simulink library "thc"  (R2021b)
settings: Solver=VariableStepAuto  StartTime=0.0  StopTime=10.0  RelTol=1e-3
undefined symbols (not defined in the file or in its folder): ATHC_APTCQA_X_C, ATHC_APTCQB_X_C, ATHC_dAy_X_C, ATHC_Qeq_X_kmh, ATHC_VbaseC_X_C, ATHC_VbaseC_Y_W, ATHC_VbaseD_X_C, ATHC_VbaseH_X_C, FALSE, KTHC_ACMaxMinT_sec, KTHC_aDeice_K, KTHC_AGSDefLv_K, KTHC_AGSLv1_K, KTHC_AGSLv2_K, KTHC_AGSLv3_K, KTHC_AGSLv4_K, KTHC_AGSLv5_K, KTHC_AirIntUpdateT_sec, KTHC_APTCOneZoneMax_W, KTHC_APTCQMaxC_W, KTHC_APTCQminC_W, KTHC_APTCQminD_W, KTHC_APTCQminRe1_W, KTHC_APTCQminRe_W, KTHC_APTCQoffT_cnt, KTHC_APTCQonT_cnt, KTHC_APTCRiLeMaxDff_W, KTHC_APTCRiLeMinDff_W, KTHC_BatInTempDef_C, KTHC_bDeice_K, KTHC_CompMaxDeice_rpm, KTHC_CompMinDeice_rpm, KTHC_CompSotxvOp_K, KTHC_CompSotxvOpLow_rpm, KTHC_CompSpdmax_rpm, KTHC_CompSpdmaxBC1_rpm, KTHC_CompSpdmaxBC_rpm, KTHC_CompSpdmid1_rpm, KTHC_CompSpdmid2_rpm, KTHC_CompSpdmid3_rpm, KTHC_CompSpdmid_rpm, KTHC_CompSpdmin_rpm, KTHC_DAPTCQ1_W, KTHC_DAPTCQ2_W, KTHC_DAPTCQ3_W, KTHC_DcChSetTemp_C, KTHC_DehumidityEN_flg, KTHC_DeiceCycTime_K, KTHC_DTambSat1_C, KTHC_DTambSat2_C, KTHC_DTambsat3_C, KTHC_DTambsat4_C, KTHC_DTambSat5_C, KTHC_DTambSat_C, KTHC_DTcabin10_C, KTHC_DTCabin11_C, KTHC_DTcabin12_C, KTHC_DTcabin1_C, KTHC_DTcabin2_C, KTHC_DTcabin3_C ... (+347)
libraries: simulink x80
(part 1 of 8)
settings Model: Creator=FVT20341  LastModifiedBy=FVT22063

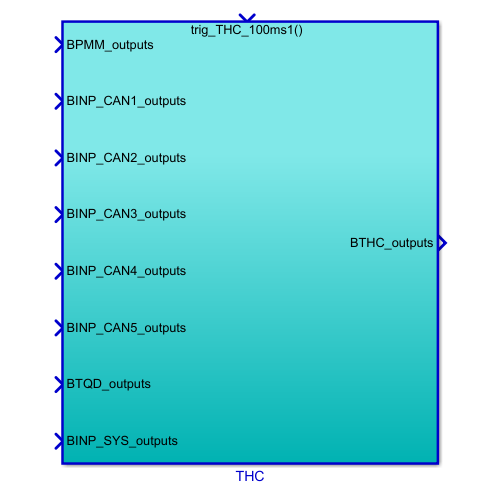
[thumbnail: Simulink's stored preview of the top-level diagram]
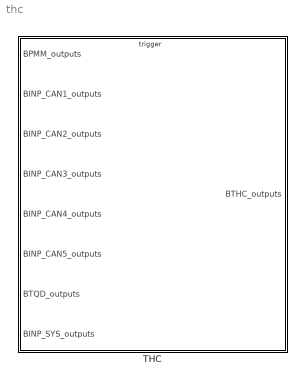
== system thc ==
  THC : Subsystem  TreatAsAtomicUnit=on
      settings: RTWSystemCode=Nonreusable function  RTWFcnNameOpts=Use subsystem name  RTWFileNameOpts=Use subsystem name

== system thc/THC ==
  BPMM_outputs : Inport  OutDataTypeStr=Bus: BPMM_outputs
  BINP_CAN1_outputs : Inport  Port=2  OutDataTypeStr=Bus: BINP_CAN1_outputs
  BINP_CAN2_outputs : Inport  Port=3  OutDataTypeStr=Bus: BINP_CAN2_outputs
  BINP_CAN3_outputs : Inport  Port=4  OutDataTypeStr=Bus: BINP_CAN3_outputs
  BINP_CAN4_outputs : Inport  Port=5  OutDataTypeStr=Bus: BINP_CAN4_outputs
  BINP_CAN5_outputs : Inport  Port=6  OutDataTypeStr=Bus: BINP_CAN5_outputs
  BTQD_outputs : Inport  Port=7  OutDataTypeStr=Bus: BTQD_outputs
  BINP_SYS_outputs : Inport  Port=8  OutDataTypeStr=Bus: BINP_SYS_outputs
  trig_THC_100ms1 : TriggerPort  TriggerType=function-call  VariantControl=(inherit)
  Bus Creator : BusCreator  Inputs=74  OutDataTypeStr=Bus: BTHC_outputs  NonVirtualBus=on
  Bus Selector : BusSelector  OutputSignals=VINP_FlashACModeMem_enum,VINP_FlashFace_flg,VINP_FlashFoot_flg,VINP_FlashFrost_flg,VINP_FlashFaceM_flg,VINP_FlashFootM_flg,VINP_FlashCCUSyncSts_flg,VINP_FlashACForceOFF_flg,VINP_FlashsigRecircSt_flg,VINP_FlashRecAutoFlg_flg,VINP_FlashAirIntenZone1M_enum,VINP_Flashfdefog_flg,VINP_FlashsigSetTempZon1St_C,VINP_FlashsigSetTempZon2StM_C
  Bus Selector1 : BusSelector  OutputSignals=VINP_VehSpeed_kph
  Bus Selector2 : BusSelector  OutputSignals=VINP_HVBMTempMax_C,VINP_HVBMTempMin_C,VINP_OBCTemp_C,VINP_DCDCTemp_C,VINP_RrTMTemp_C,VINP_RrMCUTemp_C,VINP_FrTMTemp_C,VINP_FrMCUTemp_C,VINP_ChrgPlugSta_enum,VINP_FrLLCTemp_C,VINP_RrLLCTemp_C,VINP_HVBIsoImpedenceN_Megaohm,VINP_HVBIsoImpedenceP_Megaohm,VINP_HVBHVILErr_flg
  Bus Selector3 : BusSelector  OutputSignals=VINP_PTHighTact_C,VINP_COMPStatorSpd_rpm,VINP_CompProEN_flg,VINP_PTLowP1_KPa,VINP_PTLowT1_C,VINP_PTLowP2_KPa,VINP_PTLowT2_C,VINP_PTHighP_KPa,VINP_Tamb_C,VINP_BatInTemp_C,VINP_BatOutTemp_C,VINP_MotorInTemp_C,VINP_MotorOutTemp_C,VINP_Tincar_C,VINP_SolarL_W,VINP_SolarR_W,VINP_Tevap_C,VINP_TFaceL_C,VINP_TFaceR_C,VINP_TFootL_C,VINP_TFootR_C,VINP_TFootRr_C,VINP_TFaceRr_C,VINP_EACProtectEnable_enum,VINP_TambErr_enum,VINP_SolarLErr_enum,VINP_SolarRErr_enum,VINP_TevapErr_enum,VINP_TFaceLErr_enum,VINP_TFaceRErr_enum,VINP_TFootLErr_enum,VINP_TFootRErr_enum,VINP_TFaceRrErr_enum,VINP_TFootRrErr_enum,VINP_TincarErr_enum,VINP_BatInTempErr_enum,VINP_MotorInTempErr_enum,VINP_MotorOutTempErr_enum,VINP_FanErr_enum,VINP_AGSErr_enum,VINP_EWP3Err_enum,VINP_PTHighPErr_enum,VINP_PTHighTactErr_enum,VINP_SOV1Err_enum,VINP_SOV2Err_enum,VINP_SOV3Err_enum,VINP_EXV1Err_enum,VINP_EXV2Err_enum,VINP_COMPErr_enum,VINP_BlowerErr_enum,VINP_PTLowP1Err_enum,VINP_PTLowT1Err_enum,VINP_PTLowP2Err_enum,VINP_PTLowT2Err_enum,VINP_SOTXVErr_enum,VINP_FrntPTCRearLeActHeatPwr_W,VINP_FrntPTCRearRiActHeatPwr_W,VINP_FrntPTCRiActHeatPwr_W
  Bus Selector4 : BusSelector  OutputSignals=VINP_OFFACMODE_enum,VINP_FCPFrEvtBtnACMaxReq_flg,VINP_FCPFrEvtBtnACReq_flg,VINP_FCPFrEvtBtnAutoReq_flg,VINP_FCPFrEvtBtnSyncReq_flg,VINP_sigAirIntenZon1Req_enum,VINP_sigRecircReq_flg,VINP_sigFaceReq_flg,VINP_sigFootReq_flg,VINP_sigDfrstReq_flg,VINP_sigSetTempZon1Req_C,VINP_CANMsgValidIVI2_flg,VINP_sigSetTempZon2Req_C,VINP_SmartEcoModeSW_flg
  Bus Selector5 : BusSelector  OutputSignals=VTQD_ShiftGearPosn_enum
  Bus Selector6 : BusSelector  OutputSignals=VINP_RemoteACTemp_C,VINP_RemoteAutoReq_flg
  Bus Selector7 : BusSelector  OutputSignals=VPMM_PowerSta_enum
  Ground : Ground
  Ground1 : Ground
  ThermalControl : Subsystem
  BTHC_outputs : Outport  OutDataTypeStr=Bus: BTHC_outputs
  wires:
  BPMM_outputs/1 -> Bus Selector7/1
  Bus Selector7/1 -> ThermalControl/1(VPMM_PwrSta_enum)  "<VPMM_PowerSta_enum>"
  BINP_CAN1_outputs/1 -> Bus Selector1/1
  Bus Selector1/1 -> ThermalControl/4(VINP_VehSpeed_kph)  "<VINP_VehSpeed_kph>"
  BINP_CAN3_outputs/1 -> Bus Selector2/1
  Bus Selector2/3 -> ThermalControl/7(VINP_OBCTemp_C)  "<VINP_OBCTemp_C>"
  Bus Selector2/4 -> ThermalControl/8(VINP_DCDCTemp_C)  "<VINP_DCDCTemp_C>"
  Bus Selector2/2 -> ThermalControl/6(VINP_HVBMTempMin_C)  "<VINP_HVBMTempMin_C>"
  Bus Selector2/5 -> ThermalControl/9(VINP_RrTMTemp_C)  "<VINP_RrTMTemp_C>"
  Bus Selector2/1 -> ThermalControl/5(VINP_HVBMTempMax_C)  "<VINP_HVBMTempMax_C>"
  Bus Selector2/6 -> ThermalControl/10(VINP_RrMCUTemp_C)  "<VINP_RrMCUTemp_C>"
  Bus Selector2/7 -> ThermalControl/11(VINP_FrTMTemp_C)  "<VINP_FrTMTemp_C>"
  Bus Selector2/8 -> ThermalControl/12(VINP_FrMCUTemp_C)  "<VINP_FrMCUTemp_C>"
  ThermalControl/32(VTHC_sigClntTHvBattOut_C) -> Bus Creator/32  "VTHC_sigClntTHvBattOut_C"
  ThermalControl/31(VTHC_sigSetTempZon2St_C) -> Bus Creator/31  "VTHC_sigSetTempZon2St_C"
  ThermalControl/30(VTHC_sigSetTempZon1St_C) -> Bus Creator/30  "VTHC_sigSetTempZon1St_C"
  ThermalControl/29(VTHC_sigRecircSt_flg) -> Bus Creator/29  "VTHC_sigRecircSt_flg"
  ThermalControl/28(VTHC_sigWindDirZon1St_enum) -> Bus Creator/28  "VTHC_sigWindDirZon1St_enum"
  ThermalControl/27(VTHC_sigAirIntenZon1St_enum) -> Bus Creator/27  "VTHC_sigAirIntenZon1St_enum"
  ThermalControl/26(VTHC_CCUSyncLampSts_flg) -> Bus Creator/26  "VTHC_CCUSyncLampSts_flg"
  ThermalControl/25(VTHC_CCUACMaxLampSts_flg) -> Bus Creator/25  "VTHC_CCUACMaxLampSts_flg"
  ThermalControl/24(VTHC_CCUAutoLampSts_flg) -> Bus Creator/24  "VTHC_CCUAutoLampSts_flg"
  ThermalControl/23(VTHC_CCUACLampSts_flg) -> Bus Creator/23  "VTHC_CCUACLampSts_flg"
  ThermalControl/22(VTHC_CabinMode_enum) -> Bus Creator/22  "VTHC_CabinMode_enum"
  ThermalControl/21(VTHC_EDriveMode_enum) -> Bus Creator/21  "VTHC_EDriveMode_enum"
  ThermalControl/20(VTHC_BatteryMode_enum) -> Bus Creator/20  "VTHC_BatteryMode_enum"
  ThermalControl/19(VTHC_FDBlowerCmd_pct) -> Bus Creator/19  "VTHC_FDBlowerCmd_pct"
  ThermalControl/17(VTHC_FDFrRiAPTCHeatPwrCmd_W) -> Bus Creator/17  "VTHC_FDFrRiAPTCHeatPwrCmd_W"
  ThermalControl/18(VTHC_FDRrAPTCHeatPwrCmd_W) -> Bus Creator/18  "VTHC_FDRrAPTCHeatPwrCmd_W"
  ThermalControl/16(VTHC_FDFrLeAPTCHeatPwrCmd_W) -> Bus Creator/16  "VTHC_FDFrLeAPTCHeatPwrCmd_W"
  ThermalControl/15(VTHC_FDEWP3Cmd_enum) -> Bus Creator/15  "VTHC_FDEWP3Cmd_enum"
  ThermalControl/14(VTHC_FDEWP2Cmd_enum) -> Bus Creator/14  "VTHC_FDEWP2Cmd_enum"
  ThermalControl/13(VTHC_FDEWP1Cmd_enum) -> Bus Creator/13  "VTHC_FDEWP1Cmd_enum"
  ThermalControl/12(VTHC_FDAGSCmd_enum) -> Bus Creator/12  "VTHC_FDAGSCmd_enum"
  ThermalControl/11(VTHC_CoolgFanActDuty_pct) -> Bus Creator/11  "VTHC_CoolgFanActDuty_pct"
  ThermalControl/10(VTHC_FDFrWPTCHeatPwrCmd_W) -> Bus Creator/10  "VTHC_FDFrWPTCHeatPwrCmd_W"
  ThermalControl/9(VTHC_FDTWVCmd_pct) -> Bus Creator/9  "VTHC_FDTWVCmd_pct"
  ThermalControl/8(VTHC_FDFWVCmd_flg) -> Bus Creator/8  "VTHC_FDFWVCmd_flg"
  ThermalControl/7(VTHC_FDSOTXVCmd_flg) -> Bus Creator/7  "VTHC_FDSOTXVCmd_flg"
  ThermalControl/6(VTHC_FDEXV2Cmd_step) -> Bus Creator/6  "VTHC_FDEXV2Cmd_step"
  ThermalControl/5(VTHC_FDEXV1Cmd_step) -> Bus Creator/5  "VTHC_FDEXV1Cmd_step"
  ThermalControl/4(VTHC_FDSOV3Cmd_flg) -> Bus Creator/4  "VTHC_FDSOV3Cmd_flg"
  ThermalControl/3(VTHC_FDSOV2Cmd_flg) -> Bus Creator/3  "VTHC_FDSOV2Cmd_flg"
  ThermalControl/2(VTHC_FDSOV1Cmd_flg) -> Bus Creator/2  "VTHC_FDSOV1Cmd_flg"
  ThermalControl/1(VTHC_FDCompCmd_rpm) -> Bus Creator/1  "VTHC_FDCompCmd_rpm"
  Bus Creator/1 -> BTHC_outputs/1  "BTHC_outputs"
  BINP_CAN4_outputs/1 -> Bus Selector3/1  "BINP_CAN4_outputs"
  Bus Selector3/4 -> ThermalControl/22(VINP_PTLowP1_kPa)  "<VINP_PTLowP1_KPa>"
  Bus Selector3/5 -> ThermalControl/23(VINP_PTLowT1_C)  "<VINP_PTLowT1_C>"
  Bus Selector3/6 -> ThermalControl/24(VINP_PTLowP2_kPa)  "<VINP_PTLowP2_KPa>"
  Bus Selector3/7 -> ThermalControl/25(VINP_PTLowT2_C)  "<VINP_PTLowT2_C>"
  Bus Selector3/8 -> ThermalControl/26(VINP_PTHighP_kPa)  "<VINP_PTHighP_KPa>"
  Bus Selector3/9 -> ThermalControl/27(VINP_Tamb_C)  "<VINP_Tamb_C>"
  Bus Selector3/10 -> ThermalControl/28(VINP_BatInTemp_C)  "<VINP_BatInTemp_C>"
  Bus Selector3/11 -> ThermalControl/29(VINP_BatOutTemp_C)  "<VINP_BatOutTemp_C>"
  Bus Selector3/12 -> ThermalControl/30(VINP_MotorInTemp_C)  "<VINP_MotorInTemp_C>"
  Bus Selector3/13 -> ThermalControl/31(VINP_MotorOutTemp_C)  "<VINP_MotorOutTemp_C>"
  Bus Selector3/14 -> ThermalControl/32(VINP_Tincar_C)  "<VINP_Tincar_C>"
  Bus Selector3/15 -> ThermalControl/33(VINP_SolarL_W)  "<VINP_SolarL_W>"
  Bus Selector3/16 -> ThermalControl/34(VINP_SolarR_W)  "<VINP_SolarR_W>"
  Bus Selector3/17 -> ThermalControl/35(VINP_Tevap_C)  "<VINP_Tevap_C>"
  Bus Selector3/18 -> ThermalControl/36(VINP_TFaceL_C)  "<VINP_TFaceL_C>"
  Bus Selector3/19 -> ThermalControl/37(VINP_TFaceR_C)  "<VINP_TFaceR_C>"
  Bus Selector3/20 -> ThermalControl/38(VINP_TFootL_C)  "<VINP_TFootL_C>"
  Bus Selector3/21 -> ThermalControl/39(VINP_TFootR_C)  "<VINP_TFootR_C>"
  Bus Selector3/22 -> ThermalControl/40(VINP_TFootRr_C)  "<VINP_TFootRr_C>"
  Bus Selector3/23 -> ThermalControl/41(VINP_TFaceRr_C)  "<VINP_TFaceRr_C>"
  BINP_CAN2_outputs/1 -> Bus Selector4/1  "BINP_CAN2_outputs"
  Bus Selector4/2 -> ThermalControl/78(VINP_FCPFrEvtBtnACMaxReq_flg)  "<VINP_FCPFrEvtBtnACMaxReq_flg>"
  Bus Selector4/3 -> ThermalControl/79(VINP_FCPFrEvtBtnACReq_flg)  "<VINP_FCPFrEvtBtnACReq_flg>"
  Bus Selector4/4 -> ThermalControl/80(VINP_FCPFrEvtBtnAutoReq_flg)  "<VINP_FCPFrEvtBtnAutoReq_flg>"
  Bus Selector4/5 -> ThermalControl/81(VINP_FCPFrEvtBtnSyncReq_flg)  "<VINP_FCPFrEvtBtnSyncReq_flg>"
  Bus Selector4/6 -> ThermalControl/82(VINP_sigAirIntenZon1Req_enum)  "<VINP_sigAirIntenZon1Req_enum>"
  Bus Selector4/7 -> ThermalControl/83(VINP_sigRecircReq_flg)  "<VINP_sigRecircReq_flg>"
  Bus Selector4/8 -> ThermalControl/84(VINP_sigFaceReq_flg)  "<VINP_sigFaceReq_flg>"
  Bus Selector4/9 -> ThermalControl/85(VINP_sigFootReq_flg)  "<VINP_sigFootReq_flg>"
  Bus Selector4/10 -> ThermalControl/86(VINP_sigFrostReq_flg)  "<VINP_sigDfrstReq_flg>"
  Bus Selector4/11 -> ThermalControl/87(VINP_sigSetTempZon1Req_C)  "<VINP_sigSetTempZon1Req_C>"
  Bus Selector4/12 -> ThermalControl/88(VINP_CANMsgValidIVI2_flg)  "<VINP_CANMsgValidIVI2_flg>"
  Bus Selector4/13 -> ThermalControl/89(VINP_sigSetTempZon2Req_C)  "<VINP_sigSetTempZon2Req_C>"
  Bus Selector2/9 -> ThermalControl/13(VINP_ChrgPlugSta_enum)  "<VINP_ChrgPlugSta_enum>"
  Bus Selector3/2 -> ThermalControl/20(VINP_COMP_StatorSpd_RPM)  "<VINP_COMPStatorSpd_rpm>"
  Bus Selector3/3 -> ThermalControl/21(VINP_CompProEN_flg)  "<VINP_CompProEN_flg>"
  ThermalControl/33(VTHC_sigCbnSolarLeft_W) -> Bus Creator/33  "VTHC_sigCbnSolarLeft_W"
  ThermalControl/34(VTHC_sigClntTHvBattIn_C) -> Bus Creator/34  "VTHC_sigClntTHvBattIn_C"
  ThermalControl/35(VTHC_sigCbnSolarRight_W) -> Bus Creator/35  "VTHC_sigCbnSolarRight_W"
  ThermalControl/36(VTHC_sigAmbAirT_C) -> Bus Creator/36  "VTHC_sigAmbAirT_C"
  ThermalControl/37(VTHC_sigCbnAirT_C) -> Bus Creator/37  "VTHC_sigCbnAirT_C"
  ThermalControl/38(VTHC_ACSubMode_enum) -> Bus Creator/38  "VTHC_ACSubMode_enum"
  ThermalControl/40(VTHC_CompP_K) -> Bus Creator/40  "VTHC_CompP_K"
  ThermalControl/41(VTHC_CompI_K) -> Bus Creator/41  "VTHC_CompI_K"
  ThermalControl/42(VTHC_CompU_K) -> Bus Creator/42  "VTHC_CompU_K"
  ThermalControl/43(VTHC_CompDeltaU_K) -> Bus Creator/43  "VTHC_CompDeltaU_K"
  ThermalControl/44(VTHC_Compe_K) -> Bus Creator/44  "VTHC_Compe_K"
  ThermalControl/45(VTHC_Blowere_K) -> Bus Creator/45  "VTHC_Blowere_K"
  ThermalControl/46(VTHC_BlowerP_K) -> Bus Creator/46  "VTHC_BlowerP_K"
  ThermalControl/47(VTHC_BlowerU_K) -> Bus Creator/47  "VTHC_BlowerU_K"
  ThermalControl/48(VTHC_Vbase_pct) -> Bus Creator/48  "VTHC_Vbase_pct"
  ThermalControl/49(VTHC_BlowerI_K) -> Bus Creator/49  "VTHC_BlowerI_K"
  ThermalControl/50(VTHC_EXV2P_K) -> Bus Creator/50  "VTHC_EXV2P_K"
  ThermalControl/51(VTHC_EXV2I_K) -> Bus Creator/51  "VTHC_EXV2I_K"
  ThermalControl/52(VTHC_EXV2U_K) -> Bus Creator/52  "VTHC_EXV2U_K"
  ThermalControl/53(VTHC_EXV2e_K) -> Bus Creator/53  "VTHC_EXV2e_K"
  ThermalControl/54(VTHC_APTCP_K) -> Bus Creator/54  "VTHC_APTCP_K"
  ThermalControl/55(VTHC_APTCI_K) -> Bus Creator/55  "VTHC_APTCI_K"
  ThermalControl/56(VTHC_APTCU_K) -> Bus Creator/56  "VTHC_APTCU_K"
  ThermalControl/57(VTHC_APTCe_K) -> Bus Creator/57  "VTHC_APTCe_K"
  ThermalControl/58(VTHC_EXV1P_K) -> Bus Creator/58  "VTHC_EXV1P_K"
  ThermalControl/59(VTHC_EXV1I_K) -> Bus Creator/59  "VTHC_EXV1I_K"
  ThermalControl/60(VTHC_EXV1U_K) -> Bus Creator/60  "VTHC_EXV1U_K"
  ThermalControl/61(VTHC_EXV1e_K) -> Bus Creator/61  "VTHC_EXV1e_K"
  BTQD_outputs/1 -> Bus Selector5/1
  Bus Selector5/1 -> ThermalControl/2(VTQD_ShiftGearPosn_enum)  "<VTQD_ShiftGearPosn_enum>"
  Bus Selector3/1 -> ThermalControl/19(VINP_PTHighTact_C)  "<VINP_PTHighTact_C>"
  Bus Selector2/10 -> ThermalControl/14(VINP_FrLLCTemp_C)  "<VINP_FrLLCTemp_C>"
  Bus Selector2/11 -> ThermalControl/15(VINP_RrLLCTemp_C)  "<VINP_RrLLCTemp_C>"
  Ground/1 -> ThermalControl/3(VSCP_AGSCloseSta_flg)
  Bus Selector4/1 -> ThermalControl/77(VINP_OFFACMODE_enum)  "<VINP_OFFACMODE_enum>"
  ThermalControl/39(VTHC_FDRecyAutoCmd_enum) -> Bus Creator/39  "VTHC_FDRecyAutoCmd_enum"
  Bus Selector3/24 -> ThermalControl/42(VINP_EACProtectEnable_enum)  "<VINP_EACProtectEnable_enum>"
  Bus Selector3/25 -> ThermalControl/43(Tamb_Err)  "<VINP_TambErr_enum>"
  Bus Selector3/26 -> ThermalControl/44(SolarL_Err)  "<VINP_SolarLErr_enum>"
  Bus Selector3/27 -> ThermalControl/45(SolarR_Err)  "<VINP_SolarRErr_enum>"
  Bus Selector3/28 -> ThermalControl/46(Tevap_Err)  "<VINP_TevapErr_enum>"
  Bus Selector3/29 -> ThermalControl/47(T_Face_L_Err)  "<VINP_TFaceLErr_enum>"
  Bus Selector3/30 -> ThermalControl/48(T_Face_R_Err)  "<VINP_TFaceRErr_enum>"
  Bus Selector3/31 -> ThermalControl/49(T_Foot_L_Err)  "<VINP_TFootLErr_enum>"
  Bus Selector3/32 -> ThermalControl/50(T_Foot_R_Err)  "<VINP_TFootRErr_enum>"
  Bus Selector3/33 -> ThermalControl/51(T_Face_Rr_Err)  "<VINP_TFaceRrErr_enum>"
  Bus Selector3/34 -> ThermalControl/52(T_Foot_Rr_Err)  "<VINP_TFootRrErr_enum>"
  Bus Selector3/35 -> ThermalControl/53(Tincar_Err)  "<VINP_TincarErr_enum>"
  Bus Selector3/36 -> ThermalControl/54(Bat_In_Temp_Err)  "<VINP_BatInTempErr_enum>"
  Bus Selector3/37 -> ThermalControl/55(Motor_In_Temp_Err)  "<VINP_MotorInTempErr_enum>"
  Bus Selector3/38 -> ThermalControl/56(Motor_Out_Temp_Err)  "<VINP_MotorOutTempErr_enum>"
  Bus Selector3/39 -> ThermalControl/57(Fan_Err)  "<VINP_FanErr_enum>"
  Bus Selector3/40 -> ThermalControl/58(AGS_Err)  "<VINP_AGSErr_enum>"
  Bus Selector3/41 -> ThermalControl/59(EWP3_Err)  "<VINP_EWP3Err_enum>"
  Bus Selector3/42 -> ThermalControl/60(PT_High_P_Err)  "<VINP_PTHighPErr_enum>"
  Bus Selector3/43 -> ThermalControl/61(PT_High_Tact_Err)  "<VINP_PTHighTactErr_enum>"
  Bus Selector3/44 -> ThermalControl/62(SOV1_Err)  "<VINP_SOV1Err_enum>"
  Bus Selector3/45 -> ThermalControl/63(SOV2_Err)  "<VINP_SOV2Err_enum>"
  Bus Selector3/46 -> ThermalControl/64(SOV3_Err)  "<VINP_SOV3Err_enum>"
  Bus Selector3/47 -> ThermalControl/65(EXV1_Err)  "<VINP_EXV1Err_enum>"
  Bus Selector3/48 -> ThermalControl/66(EXV2_Err)  "<VINP_EXV2Err_enum>"
  Bus Selector3/49 -> ThermalControl/67(Comp_Err)  "<VINP_COMPErr_enum>"
  Bus Selector3/50 -> ThermalControl/68(Blower_Err)  "<VINP_BlowerErr_enum>"
  Bus Selector3/51 -> ThermalControl/69(PT_Low_P1_Err)  "<VINP_PTLowP1Err_enum>"
  Bus Selector3/52 -> ThermalControl/70(PT_Low_T1_Err)  "<VINP_PTLowT1Err_enum>"
  Bus Selector3/53 -> ThermalControl/71(PT_Low_P2_Err)  "<VINP_PTLowP2Err_enum>"
  Bus Selector3/54 -> ThermalControl/72(PT_Low_T2_Err)  "<VINP_PTLowT2Err_enum>"
  Bus Selector3/55 -> ThermalControl/73(SOTXV_Err)  "<VINP_SOTXVErr_enum>"
  ThermalControl/62(VTHC_ACModeMem_enum) -> Bus Creator/62  "VTHC_ACModeMem_enum"
  ThermalControl/63(VTHC_Face_flg) -> Bus Creator/63  "VTHC_Face_flg"
  ThermalControl/64(VTHC_Foot_flg) -> Bus Creator/64  "VTHC_Foot_flg"
  ThermalControl/65(VTHC_Frost_flg) -> Bus Creator/65  "VTHC_Frost_flg"
  ThermalControl/66(VTHC_FaceM_flg) -> Bus Creator/66  "VTHC_FaceM_flg"
  ThermalControl/67(VTHC_FootM_flg) -> Bus Creator/67  "VTHC_FootM_flg"
  ThermalControl/68(VTHC_CCUSyncSts_flg) -> Bus Creator/68  "VTHC_CCUSyncSts_flg"
  ThermalControl/69(VTHC_ACForceOFF_flg) -> Bus Creator/69  "VTHC_ACForceOFF_flg"
  ThermalControl/70(VTHC_RecAutoFlg_flg) -> Bus Creator/70  "VTHC_RecAutoFlg_flg"
  ThermalControl/71(VTHC_AirIntenZone1M_enum) -> Bus Creator/71  "VTHC_AirIntenZone1M_enum"
  ThermalControl/72(VTHC_fdefog_flg) -> Bus Creator/72  "VTHC_fdefog_flg"
  BINP_SYS_outputs/1 -> Bus Selector/1  "BINP_SYS_output"
  Bus Selector/3 -> ThermalControl/94(EEP_Foot)  "<VINP_FlashFoot_flg>"
  Bus Selector/2 -> ThermalControl/93(EEP_Face)  "<VINP_FlashFace_flg>"
  Bus Selector/4 -> ThermalControl/95(EEP_Frost)  "<VINP_FlashFrost_flg>"
  Bus Selector/1 -> ThermalControl/92(EEP_ACModeMem)  "<VINP_FlashACModeMem_enum>"
  Bus Selector/5 -> ThermalControl/96(EEP_FaceM)  "<VINP_FlashFaceM_flg>"
  Bus Selector/6 -> ThermalControl/97(EEP_FootM)  "<VINP_FlashFootM_flg>"
  Bus Selector/7 -> ThermalControl/98(EEP_CCUSyncSts)  "<VINP_FlashCCUSyncSts_flg>"
  Bus Selector/8 -> ThermalControl/99(EEP_ACForceOFF)  "<VINP_FlashACForceOFF_flg>"
  Bus Selector/9 -> ThermalControl/100(EEP_sigRecircSt)  "<VINP_FlashsigRecircSt_flg>"
  Bus Selector/10 -> ThermalControl/101(EEP_RecAutoFlg)  "<VINP_FlashRecAutoFlg_flg>"
  Bus Selector/11 -> ThermalControl/102(EEP_AirIntenZone1iM)  "<VINP_FlashAirIntenZone1M_enum>"
  Bus Selector/12 -> ThermalControl/103(EEP_fdefog)  "<VINP_Flashfdefog_flg>"
  ThermalControl/73(VTHC_sigSetTempZon2StM_C) -> Bus Creator/73
  Bus Selector/13 -> ThermalControl/104(EEP_sigSetTempZon1St)  "<VINP_FlashsigSetTempZon1St_C>"
  Bus Selector/14 -> ThermalControl/105(EEP_sigSetTempZon2StM)  "<VINP_FlashsigSetTempZon2StM_C>"
  Ground1/1 -> ThermalControl/91(ECOSW)
  BINP_CAN5_outputs/1 -> Bus Selector6/1
  Bus Selector6/2 -> ThermalControl/107(VINP_RemoteAutoReq_flg)  "<VINP_RemoteAutoReq_flg>"
  Bus Selector6/1 -> ThermalControl/106(VINP_RemoteACTemp_C)  "<VINP_RemoteACTemp_C>"
  Bus Selector4/14 -> ThermalControl/90(VINP_SmartEcoModeSW_flg)  "<VINP_SmartEcoModeSW_flg>"
  Bus Selector2/12 -> ThermalControl/16(VINP_HVBIsoImpedenceN_Mohm)  "<VINP_HVBIsoImpedenceN_Megaohm>"
  Bus Selector2/13 -> ThermalControl/17(VINP_HVBIsoImpedenceP_Mohm)  "<VINP_HVBIsoImpedenceP_Megaohm>"
  Bus Selector2/14 -> ThermalControl/18(VINP_HVBHVILErr_flg)  "<VINP_HVBHVILErr_flg>"
  Bus Selector3/56 -> ThermalControl/74(VINP_FrntPTCRearLeActHeatPwr_W)  "<VINP_FrntPTCRearLeActHeatPwr_W>"
  Bus Selector3/57 -> ThermalControl/75(VINP_FrntPTCRearRiActHeatPwr_W)  "<VINP_FrntPTCRearRiActHeatPwr_W>"
  Bus Selector3/58 -> ThermalControl/76(VINP_FrntPTCRiActHeatPwr_W)  "<VINP_FrntPTCRiActHeatPwr_W>"
  ThermalControl/74(VTHC_FDCTHCMAPTCWarningSta_flg) -> Bus Creator/74

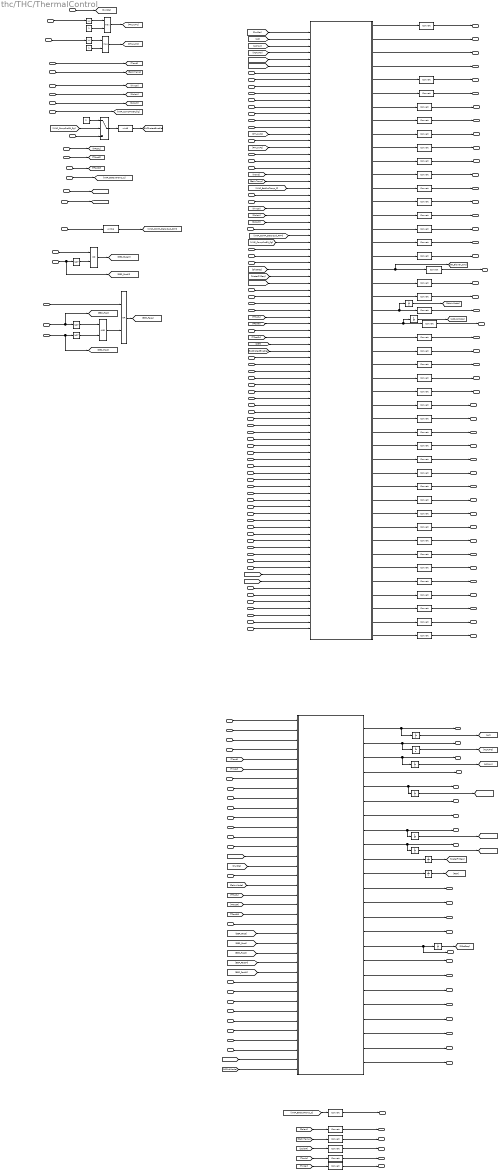
== system thc/THC/ThermalControl ==
  note: Ver Infomation
      | THCM Model V78A
      | ACHMI Model V22A
  VPMM_PwrSta_enum : Inport
  VTQD_ShiftGearPosn_enum : Inport  Port=2
  VSCP_AGSCloseSta_flg : Inport  Port=3
  VINP_VehSpeed_kph : Inport  Port=4
  VINP_HVBMTempMax_C : Inport  Port=5
  VINP_HVBMTempMin_C : Inport  Port=6
  VINP_OBCTemp_C : Inport  Port=7
  VINP_DCDCTemp_C : Inport  Port=8
  VINP_RrTMTemp_C : Inport  Port=9
  VINP_RrMCUTemp_C : Inport  Port=10
  VINP_FrTMTemp_C : Inport  Port=11
  VINP_FrMCUTemp_C : Inport  Port=12
  VINP_ChrgPlugSta_enum : Inport  Port=13
  VINP_FrLLCTemp_C : Inport  Port=14
  VINP_RrLLCTemp_C : Inport  Port=15
  VINP_HVBIsoImpedenceN_Mohm : Inport  Port=16
  VINP_HVBIsoImpedenceP_Mohm : Inport  Port=17
  VINP_HVBHVILErr_flg : Inport  Port=18
  VINP_PTHighTact_C : Inport  Port=19
  VINP_COMP_StatorSpd_RPM : Inport  Port=20
  VINP_CompProEN_flg : Inport  Port=21
  VINP_PTLowP1_kPa : Inport  Port=22
  VINP_PTLowT1_C : Inport  Port=23
  VINP_PTLowP2_kPa : Inport  Port=24
  VINP_PTLowT2_C : Inport  Port=25
  VINP_PTHighP_kPa : Inport  Port=26
  VINP_Tamb_C : Inport  Port=27
  VINP_BatInTemp_C : Inport  Port=28
  VINP_BatOutTemp_C : Inport  Port=29
  VINP_MotorInTemp_C : Inport  Port=30
  VINP_MotorOutTemp_C : Inport  Port=31
  VINP_Tincar_C : Inport  Port=32
  VINP_SolarL_W : Inport  Port=33
  VINP_SolarR_W : Inport  Port=34
  VINP_Tevap_C : Inport  Port=35
  VINP_TFaceL_C : Inport  Port=36
  VINP_TFaceR_C : Inport  Port=37
  VINP_TFootL_C : Inport  Port=38
  VINP_TFootR_C : Inport  Port=39
  VINP_TFootRr_C : Inport  Port=40
  VINP_TFaceRr_C : Inport  Port=41
  VINP_EACProtectEnable_enum : Inport  Port=42
  Tamb_Err : Inport  Port=43
  SolarL_Err : Inport  Port=44
  SolarR_Err : Inport  Port=45
  Tevap_Err : Inport  Port=46
  T_Face_L_Err : Inport  Port=47
  T_Face_R_Err : Inport  Port=48
  T_Foot_L_Err : Inport  Port=49
  T_Foot_R_Err : Inport  Port=50
  T_Face_Rr_Err : Inport  Port=51
  T_Foot_Rr_Err : Inport  Port=52
  Tincar_Err : Inport  Port=53
  Bat_In_Temp_Err : Inport  Port=54
  Motor_In_Temp_Err : Inport  Port=55
  Motor_Out_Temp_Err : Inport  Port=56
  Fan_Err : Inport  Port=57
  AGS_Err : Inport  Port=58
  EWP3_Err : Inport  Port=59
  PT_High_P_Err : Inport  Port=60
  PT_High_Tact_Err : Inport  Port=61
  SOV1_Err : Inport  Port=62
  SOV2_Err : Inport  Port=63
  SOV3_Err : Inport  Port=64
  EXV1_Err : Inport  Port=65
  EXV2_Err : Inport  Port=66
  Comp_Err : Inport  Port=67
  Blower_Err : Inport  Port=68
  PT_Low_P1_Err : Inport  Port=69
  PT_Low_T1_Err : Inport  Port=70
  PT_Low_P2_Err : Inport  Port=71
  PT_Low_T2_Err : Inport  Port=72
  SOTXV_Err : Inport  Port=73
  VINP_FrntPTCRearLeActHeatPwr_W : Inport  Port=74
  VINP_FrntPTCRearRiActHeatPwr_W : Inport  Port=75
  VINP_FrntPTCRiActHeatPwr_W : Inport  Port=76
  VINP_OFFACMODE_enum : Inport  Port=77
  VINP_FCPFrEvtBtnACMaxReq_flg : Inport  Port=78
  VINP_FCPFrEvtBtnACReq_flg : Inport  Port=79
  VINP_FCPFrEvtBtnAutoReq_flg : Inport  Port=80
  VINP_FCPFrEvtBtnSyncReq_flg : Inport  Port=81
  VINP_sigAirIntenZon1Req_enum : Inport  Port=82
  VINP_sigRecircReq_flg : Inport  Port=83
  VINP_sigFaceReq_flg : Inport  Port=84
  VINP_sigFootReq_flg : Inport  Port=85
  VINP_sigFrostReq_flg : Inport  Port=86
  VINP_sigSetTempZon1Req_C : Inport  Port=87
  VINP_CANMsgValidIVI2_flg : Inport  Port=88
  VINP_sigSetTempZon2Req_C : Inport  Port=89
  VINP_SmartEcoModeSW_flg : Inport  Port=90
  ECOSW : Inport  Port=91
  EEP_ACModeMem : Inport  Port=92
  EEP_Face : Inport  Port=93
  EEP_Foot : Inport  Port=94
  EEP_Frost : Inport  Port=95
  EEP_FaceM : Inport  Port=96
  EEP_FootM : Inport  Port=97
  EEP_CCUSyncSts : Inport  Port=98
  EEP_ACForceOFF : Inport  Port=99
  EEP_sigRecircSt : Inport  Port=100
  EEP_RecAutoFlg : Inport  Port=101
  EEP_AirIntenZone1iM : Inport  Port=102
  EEP_fdefog : Inport  Port=103
  EEP_sigSetTempZon1St : Inport  Port=104
  EEP_sigSetTempZon2StM : Inport  Port=105
  VINP_RemoteACTemp_C : Inport  Port=106
  VINP_RemoteAutoReq_flg : Inport  Port=107
  AC : Subsystem
  Abs : Abs
  Abs1 : Abs
  Constant : Constant
  Constant1 : Constant
  Constant2 : Constant  Value=2
  Data Type Conversion{,1..47,50} (49 alike) : DataTypeConversion
  Data Type Conversion48 : DataTypeConversion  OutDataTypeStr=uint8
  Data Type Conversion49 : DataTypeConversion  OutDataTypeStr=uint16
  Logical Operator : Logic  Operator=OR  AllPortsSameDT=off  OutDataTypeStr=boolean
  Logical Operator1 : Logic  Operator=OR  AllPortsSameDT=off  OutDataTypeStr=boolean
  Logical Operator2 : Logic  AllPortsSameDT=off  OutDataTypeStr=boolean
  Logical Operator3 : Logic  Operator=NOT  AllPortsSameDT=off  OutDataTypeStr=boolean
  Logical Operator4 : Logic  Operator=NOT  AllPortsSameDT=off  OutDataTypeStr=boolean
  Logical Operator5 : Logic  Operator=NOT  AllPortsSameDT=off  OutDataTypeStr=boolean
  Max : MinMax  Function=max  Inputs=2
  Max1 : MinMax  Function=max  Inputs=2
  Switch : Switch  Criteria=u2 > Threshold
  THCM_Conctrl : Subsystem
  Unit Delay{,1..5,7..11} (11 alike) : UnitDelay  SampleTime=-1  HasFrameUpgradeWarning=on
  VTHC_FDCompCmd_rpm : Outport
  VTHC_FDSOV1Cmd_flg : Outport  Port=2
  VTHC_FDSOV2Cmd_flg : Outport  Port=3
  VTHC_FDSOV3Cmd_flg : Outport  Port=4
  VTHC_FDEXV1Cmd_step : Outport  Port=5
  VTHC_FDEXV2Cmd_step : Outport  Port=6
  VTHC_FDSOTXVCmd_flg : Outport  Port=7
  VTHC_FDFWVCmd_flg : Outport  Port=8
  VTHC_FDTWVCmd_pct : Outport  Port=9
  VTHC_FDFrWPTCHeatPwrCmd_W : Outport  Port=10
  VTHC_CoolgFanActDuty_pct : Outport  Port=11
  VTHC_FDAGSCmd_enum : Outport  Port=12
  VTHC_FDEWP1Cmd_enum : Outport  Port=13
  VTHC_FDEWP2Cmd_enum : Outport  Port=14
  VTHC_FDEWP3Cmd_enum : Outport  Port=15
  VTHC_FDFrLeAPTCHeatPwrCmd_W : Outport  Port=16
  VTHC_FDFrRiAPTCHeatPwrCmd_W : Outport  Port=17
  VTHC_FDRrAPTCHeatPwrCmd_W : Outport  Port=18
  VTHC_FDBlowerCmd_pct : Outport  Port=19
  VTHC_BatteryMode_enum : Outport  Port=20
  VTHC_EDriveMode_enum : Outport  Port=21
  VTHC_CabinMode_enum : Outport  Port=22
  VTHC_CCUACLampSts_flg : Outport  Port=23
  VTHC_CCUAutoLampSts_flg : Outport  Port=24
  VTHC_CCUACMaxLampSts_flg : Outport  Port=25
  VTHC_CCUSyncLampSts_flg : Outport  Port=26
  VTHC_sigAirIntenZon1St_enum : Outport  Port=27
  VTHC_sigWindDirZon1St_enum : Outport  Port=28
  VTHC_sigRecircSt_flg : Outport  Port=29
  VTHC_sigSetTempZon1St_C : Outport  Port=30
  VTHC_sigSetTempZon2St_C : Outport  Port=31
  VTHC_sigClntTHvBattOut_C : Outport  Port=32
  VTHC_sigCbnSolarLeft_W : Outport  Port=33
  VTHC_sigClntTHvBattIn_C : Outport  Port=34
  VTHC_sigCbnSolarRight_W : Outport  Port=35
  VTHC_sigAmbAirT_C : Outport  Port=36
  VTHC_sigCbnAirT_C : Outport  Port=37
  VTHC_ACSubMode_enum : Outport  Port=38
  VTHC_FDRecyAutoCmd_enum : Outport  Port=39
  VTHC_CompP_K : Outport  Port=40
  VTHC_CompI_K : Outport  Port=41
  VTHC_CompU_K : Outport  Port=42
  VTHC_CompDeltaU_K : Outport  Port=43
  VTHC_Compe_K : Outport  Port=44
  VTHC_Blowere_K : Outport  Port=45
  VTHC_BlowerP_K : Outport  Port=46
  VTHC_BlowerU_K : Outport  Port=47
  VTHC_Vbase_pct : Outport  Port=48
  VTHC_BlowerI_K : Outport  Port=49
  VTHC_EXV2P_K : Outport  Port=50
  VTHC_EXV2I_K : Outport  Port=51
  VTHC_EXV2U_K : Outport  Port=52
  VTHC_EXV2e_K : Outport  Port=53
  VTHC_APTCP_K : Outport  Port=54
  VTHC_APTCI_K : Outport  Port=55
  VTHC_APTCU_K : Outport  Port=56
  VTHC_APTCe_K : Outport  Port=57
  VTHC_EXV1P_K : Outport  Port=58
  VTHC_EXV1I_K : Outport  Port=59
  VTHC_EXV1U_K : Outport  Port=60
  VTHC_EXV1e_K : Outport  Port=61
  VTHC_ACModeMem_enum : Outport  Port=62
  VTHC_Face_flg : Outport  Port=63
  VTHC_Foot_flg : Outport  Port=64
  VTHC_Frost_flg : Outport  Port=65
  VTHC_FaceM_flg : Outport  Port=66
  VTHC_FootM_flg : Outport  Port=67
  VTHC_CCUSyncSts_flg : Outport  Port=68
  VTHC_ACForceOFF_flg : Outport  Port=69
  VTHC_RecAutoFlg_flg : Outport  Port=70
  VTHC_AirIntenZone1M_enum : Outport  Port=71
  VTHC_fdefog_flg : Outport  Port=72
  VTHC_sigSetTempZon2StM_C : Outport  Port=73
  VTHC_FDCTHCMAPTCWarningSta_flg : Outport  Port=74
  wires:
  AC/9(VTHC_sigSetTempZon2St_C) -> Unit Delay9/1, VTHC_sigSetTempZon2St_C/1
  AC/2(VTHC_CCUAutoLampSts_flg) -> Unit Delay2/1, VTHC_CCUAutoLampSts_flg/1
  AC/6(VTHC_sigWindDirZon1St_enum) -> VTHC_sigWindDirZon1St_enum/1
  Unit Delay3/1 -> [ACMAX]
  AC/4(VTHC_CCUSyncLampSts_flg) -> VTHC_CCUSyncLampSts_flg/1
  AC/1(VTHC_CCUACLampSts_flg) -> Unit Delay1/1, VTHC_CCUACLampSts_flg/1
  AC/5(VTHC_sigAirIntenZon1St_enum) -> Unit Delay4/1, VTHC_sigAirIntenZon1St_enum/1
  AC/8(VTHC_sigSetTempZon1St_C) -> Unit Delay5/1, VTHC_sigSetTempZon1St_C/1
  THCM_Conctrl/19(FD_Blower_Cmd) -> Data Type Conversion/1, [FD_Blower_Cmd]
  Unit Delay5/1 -> [sigSetTempZon1St]
  AC/7(VTHC_sigRecircSt_flg) -> VTHC_sigRecircSt_flg/1
  AC/3(VTHC_CCUACMaxLampSts_flg) -> Unit Delay3/1, VTHC_CCUACMaxLampSts_flg/1
  VPMM_PwrSta_enum/1 -> [PwrSta]
  THCM_Conctrl/13(FD_EWP1_Cmd) -> Data Type Conversion3/1
  THCM_Conctrl/11(CoolgFanActDuty) -> Data Type Conversion1/1
  THCM_Conctrl/18(FD_RrAPTCHeatPwr_Cmd) -> Data Type Conversion8/1
  THCM_Conctrl/21(EDriveMode) -> Data Type Conversion22/1
  THCM_Conctrl/20(BatteryMode) -> Data Type Conversion21/1
  THCM_Conctrl/16(FD_FrLeAPTCHeatPwr_Cmd) -> Data Type Conversion6/1
  VINP_Tincar_C/1 -> [Tincar]
  THCM_Conctrl/9(FD_TWV_Cmd) -> Data Type Conversion19/1
  THCM_Conctrl/4(FD_SOV3_Cmd) -> VTHC_FDSOV3Cmd_flg/1
  VINP_SolarR_W/1 -> [SolarR]
  THCM_Conctrl/15(FD_EWP3_Cmd) -> Data Type Conversion5/1
  THCM_Conctrl/2(FD_SOV1_Cmd) -> VTHC_FDSOV1Cmd_flg/1
  Unit Delay2/1 -> [ACAUTO]
  THCM_Conctrl/7(FD_SOTXV_Cmd) -> Data Type Conversion46/1
  THCM_Conctrl/14(FD_EWP2_Cmd) -> Data Type Conversion4/1
  THCM_Conctrl/3(FD_SOV2_Cmd) -> VTHC_FDSOV2Cmd_flg/1
  THCM_Conctrl/6(FD_EXV2_Cmd) -> Data Type Conversion17/1
  VINP_Tamb_C/1 -> [Tamb]
  THCM_Conctrl/8(FD_FWV_Cmd) -> Data Type Conversion18/1
  VINP_BatInTemp_C/1 -> [BatInTemp]
  Unit Delay1/1 -> [AC]
  THCM_Conctrl/17(FD_FrRiAPTCHeatPwr_Cmd) -> Data Type Conversion7/1
  VINP_SolarL_W/1 -> [SolarL]
  THCM_Conctrl/12(FD_AGS_Cmd) -> Data Type Conversion2/1
  VINP_TFootL_C/1 -> [TFootL]
  Unit Delay4/1 -> [sigAirIntenZon1St]
  THCM_Conctrl/10(FD_FrWPTCHeatPwr_Cmd) -> Data Type Conversion20/1
  THCM_Conctrl/22(CabinMode) -> Unit Delay11/1, Data Type Conversion23/1
  [SolarL] -> Data Type Conversion41/1  "VTHC_sigCbnSolarLeft_W"
  [SolarR] -> Data Type Conversion43/1  "VTHC_sigCbnSolarRight_W"
  [BatInTemp] -> Data Type Conversion42/1  "VTHC_sigClntTHvBattIn_C"
  [Tamb] -> Data Type Conversion44/1  "VTHC_sigAmbAirT_C"
  [Tincar] -> Data Type Conversion45/1  "VTHC_sigCbnAirT_C"
  VINP_PTLowP2_kPa/1 -> Abs/1
  Abs/1 -> Max/1
  Constant/1 -> Max/2
  Constant1/1 -> Max1/2
  Abs1/1 -> Max1/1
  VINP_PTLowP1_kPa/1 -> Abs1/1
  VINP_TFootR_C/1 -> [TFootR]
  VINP_TFootRr_C/1 -> [TFootRr]
  VINP_CompProEN_flg/1 -> [VINP_CompProEN_flg]
  THCM_Conctrl/23(ACSubMode) -> Data Type Conversion28/1, Unit Delay/1
  THCM_Conctrl/24(VTHC_CompP_K) -> Data Type Conversion29/1
  THCM_Conctrl/25(VTHC_CompI_K) -> Data Type Conversion35/1
  THCM_Conctrl/26(VTHC_CompU_K) -> Data Type Conversion36/1
  THCM_Conctrl/27(VTHC_CompDeltaU_K) -> Data Type Conversion34/1
  THCM_Conctrl/28(VTHC_Compe_K) -> Data Type Conversion33/1
  THCM_Conctrl/29(VTHC_Blowere_K) -> Data Type Conversion32/1
  THCM_Conctrl/30(VTHC_BlowerP_K) -> Data Type Conversion31/1
  THCM_Conctrl/31(VTHC_BlowerU_K) -> Data Type Conversion30/1
  THCM_Conctrl/32(VTHC_Vbase_pct) -> Data Type Conversion37/1
  THCM_Conctrl/33(VTHC_BlowerI_K) -> Data Type Conversion38/1
  THCM_Conctrl/34(VTHC_EXV2P_K) -> Data Type Conversion24/1
  THCM_Conctrl/35(VTHC_EXV2I_K) -> Data Type Conversion25/1
  THCM_Conctrl/36(VTHC_EXV2U_K) -> Data Type Conversion26/1
  THCM_Conctrl/37(VTHC_EXV2e_K) -> Data Type Conversion27/1
  THCM_Conctrl/39(VTHC_APTCI_K) -> Data Type Conversion16/1
  THCM_Conctrl/40(VTHC_APTCU_K) -> Data Type Conversion15/1
  THCM_Conctrl/41(VTHC_APTCe_K) -> Data Type Conversion14/1
  THCM_Conctrl/42(VTHC_EXV1P_K) -> Data Type Conversion11/1
  THCM_Conctrl/43(VTHC_EXV1I_K) -> Data Type Conversion12/1
  THCM_Conctrl/44(VTHC_EXV1U_K) -> Data Type Conversion13/1
  THCM_Conctrl/45(VTHC_EXV1e_K) -> Data Type Conversion9/1
  THCM_Conctrl/5(FD_EXV1_Cmd) -> Data Type Conversion10/1
  Data Type Conversion1/1 -> VTHC_CoolgFanActDuty_pct/1  "CoolgFanActDuty"
  Data Type Conversion2/1 -> VTHC_FDAGSCmd_enum/1  "FD_AGS_Cmd"
  Data Type Conversion3/1 -> VTHC_FDEWP1Cmd_enum/1  "FD_EWP1_Cmd"
  Data Type Conversion4/1 -> VTHC_FDEWP2Cmd_enum/1  "FD_EWP2_Cmd"
  Data Type Conversion5/1 -> VTHC_FDEWP3Cmd_enum/1  "FD_EWP3_Cmd"
  Data Type Conversion6/1 -> VTHC_FDFrLeAPTCHeatPwrCmd_W/1  "FD_FrLeAPTCHeatPwr_Cmd"
  Data Type Conversion8/1 -> VTHC_FDRrAPTCHeatPwrCmd_W/1  "FD_RrAPTCHeatPwr_Cmd"
  Data Type Conversion7/1 -> VTHC_FDFrRiAPTCHeatPwrCmd_W/1  "FD_FrRiAPTCHeatPwr_Cmd"
  Data Type Conversion9/1 -> VTHC_EXV1e_K/1  "VTHC_EXV1e_K"
  Data Type Conversion10/1 -> VTHC_FDEXV1Cmd_step/1  "FD_EXV1_Cmd"
  Data Type Conversion11/1 -> VTHC_EXV1P_K/1  "VTHC_EXV1P_K"
  Data Type Conversion12/1 -> VTHC_EXV1I_K/1  "VTHC_EXV1I_K"
  Data Type Conversion13/1 -> VTHC_EXV1U_K/1  "VTHC_EXV1U_K"
  Data Type Conversion14/1 -> VTHC_APTCe_K/1  "VTHC_APTCe_K"
  Data Type Conversion15/1 -> VTHC_APTCU_K/1  "VTHC_APTCU_K"
  Data Type Conversion16/1 -> VTHC_APTCI_K/1  "VTHC_APTCI_K"
  THCM_Conctrl/38(VTHC_APTCP_K) -> Data Type Conversion39/1
  Data Type Conversion17/1 -> VTHC_FDEXV2Cmd_step/1  "FD_EXV2_Cmd"
  Data Type Conversion18/1 -> VTHC_FDFWVCmd_flg/1  "FD_FWV_Cmd"
  Data Type Conversion19/1 -> VTHC_FDTWVCmd_pct/1  "FD_TWV_Cmd"
  Data Type Conversion20/1 -> VTHC_FDFrWPTCHeatPwrCmd_W/1  "FD_FrWPTCHeatPwr_Cmd"
  Data Type Conversion21/1 -> VTHC_BatteryMode_enum/1  "BatteryMode"
  Data Type Conversion22/1 -> VTHC_EDriveMode_enum/1  "EDriveMode"
  Data Type Conversion23/1 -> VTHC_CabinMode_enum/1  "CabinMode"
  Data Type Conversion24/1 -> VTHC_EXV2P_K/1  "VTHC_EXV2P_K"
  Data Type Conversion25/1 -> VTHC_EXV2I_K/1  "VTHC_EXV2I_K"
  Data Type Conversion26/1 -> VTHC_EXV2U_K/1  "VTHC_EXV2U_K"
  Data Type Conversion27/1 -> VTHC_EXV2e_K/1  "VTHC_EXV2e_K"
  Data Type Conversion28/1 -> VTHC_ACSubMode_enum/1  "ACSubMode"
  Data Type Conversion29/1 -> VTHC_CompP_K/1  "VTHC_CompP_K"
  Data Type Conversion30/1 -> VTHC_BlowerU_K/1  "VTHC_BlowerU_K"
  Data Type Conversion31/1 -> VTHC_BlowerP_K/1  "VTHC_BlowerP_K"
  Data Type Conversion32/1 -> VTHC_Blowere_K/1  "VTHC_Blowere_K"
  Data Type Conversion33/1 -> VTHC_Compe_K/1  "VTHC_Compe_K"
  Data Type Conversion34/1 -> VTHC_CompDeltaU_K/1  "VTHC_CompDeltaU_K"
  Data Type Conversion35/1 -> VTHC_CompI_K/1  "VTHC_CompI_K"
  Data Type Conversion36/1 -> VTHC_CompU_K/1  "VTHC_CompU_K"
  Data Type Conversion37/1 -> VTHC_Vbase_pct/1  "VTHC_Vbase_pct"
  Data Type Conversion38/1 -> VTHC_BlowerI_K/1  "VTHC_BlowerI_K"
  Data Type Conversion39/1 -> VTHC_APTCP_K/1  "VTHC_APTCP_K"
  Data Type Conversion40/1 -> VTHC_sigClntTHvBattOut_C/1  "VINP_BatOutTemp_C"
  Data Type Conversion41/1 -> VTHC_sigCbnSolarLeft_W/1  "SolarL"
  Data Type Conversion42/1 -> VTHC_sigClntTHvBattIn_C/1  "BatInTemp"
  Data Type Conversion43/1 -> VTHC_sigCbnSolarRight_W/1  "SolarR"
  Data Type Conversion44/1 -> VTHC_sigAmbAirT_C/1  "Tamb"
  Data Type Conversion45/1 -> VTHC_sigCbnAirT_C/1  "Tincar"
  AC/10(WaterFillReq) -> Unit Delay7/1
  AC/16(Frost) -> VTHC_Frost_flg/1, Unit Delay8/1
  Unit Delay8/1 -> [DfrstReq]
  Unit Delay7/1 -> [WaterFillReq]
  Unit Delay9/1 -> [sigSetTempZon2St]
  Data Type Conversion/1 -> VTHC_FDBlowerCmd_pct/1
  Data Type Conversion46/1 -> VTHC_FDSOTXVCmd_flg/1
  VINP_BatOutTemp_C/1 -> [VINP_BatOutTemp_C]
  [VINP_BatOutTemp_C] -> Data Type Conversion40/1
  AC/11(PET) -> Unit Delay10/1
  Unit Delay10/1 -> [PET]
  THCM_Conctrl/1(FD_Comp_Cmd) -> Data Type Conversion47/1
  Data Type Conversion47/1 -> VTHC_FDCompCmd_rpm/1  "VTHC_FDCompCmd_rpm"
  Unit Delay11/1 -> [CabinMode]
  AC/12(FD_RecyAuto_Cmd) -> VTHC_FDRecyAutoCmd_enum/1
  [VINP_CompProEN_flg] -> Switch/2
  Switch/1 -> Data Type Conversion48/1
  Constant2/1 -> Switch/1
  VINP_EACProtectEnable_enum/1 -> Switch/3
  Max1/1 -> [PTLowP1]
  Max/1 -> [PTLowP2]
  [PwrSta] -> THCM_Conctrl/1(PwrSta)
  [AC] -> THCM_Conctrl/2(AC)
  [ACMAX] -> THCM_Conctrl/3(ACMax)
  [ACAUTO] -> THCM_Conctrl/4(ACAuto)
  [sigSetTempZon1St] -> THCM_Conctrl/5(sigSetTempZon1St)
  [sigAirIntenZon1St] -> THCM_Conctrl/6(sigAirIntenZon1St)
  VINP_VehSpeed_kph/1 -> THCM_Conctrl/7(VehSpeed)
  VINP_HVBMTempMax_C/1 -> THCM_Conctrl/8(HVBMTempMax)
  VINP_HVBMTempMin_C/1 -> THCM_Conctrl/9(HVBMTempMin)
  [PTLowP1] -> THCM_Conctrl/16(PT_ Low_P1)
  VINP_OBCTemp_C/1 -> THCM_Conctrl/10(OBCTemp)
  VINP_DCDCTemp_C/1 -> THCM_Conctrl/11(DCDCTemp)
  [PTLowP2] -> THCM_Conctrl/18(PT_Low_P2)
  VINP_RrTMTemp_C/1 -> THCM_Conctrl/12(Rr_TMTemp)
  VINP_RrMCUTemp_C/1 -> THCM_Conctrl/13(Rr_MCUTemp)
  VINP_FrTMTemp_C/1 -> THCM_Conctrl/14(Fr_TMTemp)
  VINP_FrMCUTemp_C/1 -> THCM_Conctrl/15(Fr_MCUTemp)
  [VINP_BatOutTemp_C] -> THCM_Conctrl/24(Bat_Out_Temp)
  [Tamb] -> THCM_Conctrl/22(Tamb)
  VINP_PTLowT1_C/1 -> THCM_Conctrl/17(PT_ Low_T1)
  [BatInTemp] -> THCM_Conctrl/23(Bat_In_Temp)
  VINP_PTLowT2_C/1 -> THCM_Conctrl/19(PT_ Low_T2)
  VINP_PTHighP_kPa/1 -> THCM_Conctrl/20(PT_High_P)
  VINP_PTHighTact_C/1 -> THCM_Conctrl/21(PT_High_Tact)
  [Tincar] -> THCM_Conctrl/27(Tincar)
  [SolarL] -> THCM_Conctrl/28(SolarL)
  [VINP_CompProEN_flg] -> THCM_Conctrl/32(CompProEN)
  [SolarR] -> THCM_Conctrl/29(SolarR)
  VINP_MotorInTemp_C/1 -> THCM_Conctrl/25(Motor_In_Temp)
  VINP_MotorOutTemp_C/1 -> THCM_Conctrl/26(Motor_Out_Temp)
  VINP_Tevap_C/1 -> THCM_Conctrl/30(Tevap)
  VINP_COMP_StatorSpd_RPM/1 -> Data Type Conversion49/1
  [DfrstReq] -> THCM_Conctrl/36(DfrstReq)
  VSCP_AGSCloseSta_flg/1 -> THCM_Conctrl/33(VSCP_AGSCloseSta_flg)
  [WaterFillReq] -> THCM_Conctrl/37(WaterFillReq)
  VTQD_ShiftGearPosn_enum/1 -> THCM_Conctrl/34(ShiftGearPosn)
  [sigSetTempZon2St] -> THCM_Conctrl/38(sigSetTempZon2St)
  VINP_ChrgPlugSta_enum/1 -> THCM_Conctrl/35(ChrgPlugSta)
  [TFootR] -> THCM_Conctrl/44(T_Foot_R)
  VINP_FrLLCTemp_C/1 -> THCM_Conctrl/39(Fr_LLCTemp)
  [TFootL] -> THCM_Conctrl/43(T_Foot_L)
  VINP_RrLLCTemp_C/1 -> THCM_Conctrl/40(Rr_LLCTemp)
  VINP_TFaceL_C/1 -> THCM_Conctrl/41(T_Face_L)
  [PET] -> THCM_Conctrl/47(PET)
  [TFootRr] -> THCM_Conctrl/46(T_Foot_Rr)
  [EACProtectEnable] -> THCM_Conctrl/48(EACProtectEnable)
  VINP_TFaceR_C/1 -> THCM_Conctrl/42(T_Face_R)
  VINP_TFaceRr_C/1 -> THCM_Conctrl/45(T_Face_Rr)
  Tamb_Err/1 -> THCM_Conctrl/49(Tamb_Err)
  SolarL_Err/1 -> THCM_Conctrl/50(SolarL_Err)
  SolarR_Err/1 -> THCM_Conctrl/51(SolarR_Err)
  Tevap_Err/1 -> THCM_Conctrl/52(Tevap_Err)
  T_Face_L_Err/1 -> THCM_Conctrl/53(T_Face_L_Err)
  T_Face_R_Err/1 -> THCM_Conctrl/54(T_Face_R_Err)
  T_Foot_L_Err/1 -> THCM_Conctrl/55(T_Foot_L_Err)
  T_Foot_R_Err/1 -> THCM_Conctrl/56(T_Foot_R_Err)
  T_Face_Rr_Err/1 -> THCM_Conctrl/57(T_Face_Rr_Err)
  T_Foot_Rr_Err/1 -> THCM_Conctrl/58(T_Foot_Rr_Err)
  Tincar_Err/1 -> THCM_Conctrl/59(Tincar_Err)
  Bat_In_Temp_Err/1 -> THCM_Conctrl/60(Bat_In_Temp_Err)
  Motor_In_Temp_Err/1 -> THCM_Conctrl/61(Motor_In_Temp_Err)
  Motor_Out_Temp_Err/1 -> THCM_Conctrl/62(Motor_Out_Temp_Err)
  Fan_Err/1 -> THCM_Conctrl/63(Fan_Err)
  AGS_Err/1 -> THCM_Conctrl/64(AGS_Err)
  EWP3_Err/1 -> THCM_Conctrl/65(EWP3_Err)
  PT_High_P_Err/1 -> THCM_Conctrl/66(PT_High_P_Err)
  PT_High_Tact_Err/1 -> THCM_Conctrl/67(PT_High_Tact_Err)
  SOV1_Err/1 -> THCM_Conctrl/68(SOV1_Err)
  SOV2_Err/1 -> THCM_Conctrl/69(SOV2_Err)
  SOV3_Err/1 -> THCM_Conctrl/70(SOV3_Err)
  EXV1_Err/1 -> THCM_Conctrl/71(EXV1_Err)
  EXV2_Err/1 -> THCM_Conctrl/72(EXV2_Err)
  Comp_Err/1 -> THCM_Conctrl/73(Comp_Err)
  Blower_Err/1 -> THCM_Conctrl/74(Blower_Err)
  PT_Low_P1_Err/1 -> THCM_Conctrl/75(PT_Low_P1_Err)
  PT_Low_T1_Err/1 -> THCM_Conctrl/76(PT_Low_T1_Err)
  PT_Low_P2_Err/1 -> THCM_Conctrl/77(PT_Low_P2_Err)
  PT_Low_T2_Err/1 -> THCM_Conctrl/78(PT_Low_T2_Err)
  SOTXV_Err/1 -> THCM_Conctrl/79(SOTXV_Err)
  VINP_FCPFrEvtBtnACMaxReq_flg/1 -> AC/1(VINP_FCPFrEvtBtnACMaxReq_flg)
  VINP_FCPFrEvtBtnACReq_flg/1 -> AC/2(VINP_FCPFrEvtBtnACReq_flg)
  [Tamb] -> AC/5(VINP_Tamb_C)
  VINP_FCPFrEvtBtnAutoReq_flg/1 -> AC/3(VINP_FCPFrEvtBtnAutoReq_flg)
  [Tincar] -> AC/6(VINP_Tincar_C)
  VINP_FCPFrEvtBtnSyncReq_flg/1 -> AC/4(VINP_FCPFrEvtBtnSyncReq_flg)
  VINP_sigAirIntenZon1Req_enum/1 -> AC/7(VINP_sigAirIntenZon1Req_enum)
  VINP_sigRecircReq_flg/1 -> AC/8(VINP_sigRecircReq_flg)
  VINP_sigFaceReq_flg/1 -> AC/9(VINP_sigFaceReq_flg)
  VINP_sigFootReq_flg/1 -> AC/10(VINP_sigFootReq_flg)
  VINP_sigFrostReq_flg/1 -> AC/11(VINP_sigFrostReq_flg)
  VINP_sigSetTempZon1Req_C/1 -> AC/12(VINP_sigSetTempZon1Req_C)
  [FD_Blower_Cmd] -> AC/15(VTHC_FDBlowerCmd_pct)
  VINP_CANMsgValidIVI2_flg/1 -> AC/13(VINP_CANMsgValidIVI2_flg)
  [PwrSta] -> AC/16(PwrSta)
  VINP_sigSetTempZon2Req_C/1 -> AC/14(VINP_sigSetTempZon2Req_C)
  [CabinMode] -> AC/18(CabinMode)
  [TFootL] -> AC/19(T_Foot_L)
  VINP_OFFACMODE_enum/1 -> AC/17(OFF_AC_MODE)
  [TFootR] -> AC/20(T_Foot_R)
  [TFootRr] -> AC/21(T_Foot_Rr)
  EEP_ACModeMem/1 -> AC/22(EEP_ACModeMem)
  AC/13(ACModeMem) -> VTHC_ACModeMem_enum/1
  AC/14(Face) -> VTHC_Face_flg/1
  AC/15(Foot) -> VTHC_Foot_flg/1
  AC/17(FaceM) -> VTHC_FaceM_flg/1
  AC/18(FootM) -> VTHC_FootM_flg/1
  AC/19(CCUSyncSts) -> VTHC_CCUSyncSts_flg/1
  AC/20(ACForceOFF) -> VTHC_ACForceOFF_flg/1
  AC/22(AirIntenZone1M) -> VTHC_AirIntenZone1M_enum/1
  AC/23(fdefog) -> VTHC_fdefog_flg/1
  EEP_CCUSyncSts/1 -> AC/28(EEP_CCUSyncSts)
  EEP_ACForceOFF/1 -> AC/29(EEP_ACForceOFF)
  EEP_sigRecircSt/1 -> AC/30(EEP_sigRecircSt)
  EEP_RecAutoFlg/1 -> AC/31(EEP_RecAutoFlg)
  EEP_AirIntenZone1iM/1 -> AC/32(EEP_AirIntenZone1M)
  EEP_fdefog/1 -> AC/33(EEP_fdefog)
  EEP_sigSetTempZon1St/1 -> AC/34(EEP_sigSetTempZon1Req)
  EEP_sigSetTempZon2StM/1 -> AC/35(EEP_sigSetTempZon2Req)
  AC/21(RecAutoFlg) -> VTHC_RecAutoFlg_flg/1
  AC/24(VTHC_sigSetTempZon2StM_C) -> VTHC_sigSetTempZon2StM_C/1
  ECOSW/1 -> THCM_Conctrl/80(ECOSW)
  VINP_RemoteACTemp_C/1 -> [RemoteACTemp]
  [RemoteACTemp] -> THCM_Conctrl/81(RemoteACTemp)
  VINP_RemoteAutoReq_flg/1 -> [RemoteAutoReq]
  [RemoteAutoReq] -> THCM_Conctrl/82(RemoteAutoReq)
  [RemoteAutoReq] -> AC/36(VINP_RemoteAutoReq_flg)
  Unit Delay/1 -> [ACSubMode]
  [ACSubMode] -> AC/37(ACSubMode)
  Data Type Conversion48/1 -> [EACProtectEnable]
  Data Type Conversion49/1 -> [VINP_COMP_StatorSpd_RPM]
  [VINP_COMP_StatorSpd_RPM] -> THCM_Conctrl/31(CompFB)
  EEP_FootM/1 -> [EEP_FootM], Logical Operator3/1
  EEP_FaceM/1 -> Logical Operator/1
  Logical Operator/1 -> [EEP_FaceM]
  [EEP_FaceM] -> AC/26(EEP_FaceM)
  [EEP_FootM] -> AC/27(EEP_FootM)
  Logical Operator5/1 -> Logical Operator2/2
  EEP_Foot/1 -> [EEP_Foot], Logical Operator4/1
  EEP_Frost/1 -> [EEP_Frost], Logical Operator5/1
  Logical Operator2/1 -> Logical Operator1/2
  EEP_Face/1 -> Logical Operator1/1
  Logical Operator1/1 -> [EEP_Face]
  [EEP_Face] -> AC/23(EEP_Face)
  [EEP_Frost] -> AC/25(EEP_Frost)
  [EEP_Foot] -> AC/24(EEP_Foot)
  Logical Operator3/1 -> Logical Operator/2
  Logical Operator4/1 -> Logical Operator2/1
  VINP_SmartEcoModeSW_flg/1 -> THCM_Conctrl/83(VINP_SmartEcoModeSW_flg)
  VINP_HVBIsoImpedenceN_Mohm/1 -> THCM_Conctrl/84(VINP_HVBIsoImpedenceN_Mohm)
  VINP_HVBIsoImpedenceP_Mohm/1 -> THCM_Conctrl/85(VINP_HVBIsoImpedenceP_Mohm)
  VINP_HVBHVILErr_flg/1 -> THCM_Conctrl/86(VINP_HVBHVILErr_flg)
  VINP_FrntPTCRearLeActHeatPwr_W/1 -> THCM_Conctrl/87(VINP_FrntPTCRearLeActHeatPwr_W)
  VINP_FrntPTCRearRiActHeatPwr_W/1 -> THCM_Conctrl/88(VINP_FrntPTCRearRiActHeatPwr_W)
  VINP_FrntPTCRiActHeatPwr_W/1 -> THCM_Conctrl/89(VINP_FrntPTCRiActHeatPwr_W)
  THCM_Conctrl/46(APTCForceOFF) -> Data Type Conversion50/1
  Data Type Conversion50/1 -> VTHC_FDCTHCMAPTCWarningSta_flg/1  "VTHC_FDCTHCMAPTCWarningSta_flg"
